simulink library "ddm"  (R2021b)
settings: Solver=VariableStepAuto  StartTime=0.0  StopTime=10.0  RelTol=1e-3
undefined symbols (not defined in the file or in its folder): ENUM_ADASACCSTA_ERROR, ENUM_ADASACCSTA_OFF, ENUM_ADASACCSTA_STANDBY, ENUM_ADASISASTA_OFF, ENUM_ALLOWMOV_ALLOWREADY, ENUM_APS, ENUM_BRKSTA_ERROR, ENUM_BRKSTA_OFF, ENUM_BRKSTA_ON, ENUM_CHGPREACTERRSTA_OBCPRE, ENUM_DCDCFAULTSTA_ANYFAULTLV1, ENUM_DCDCFAULTSTA_ANYFAULTLV2, ENUM_DRIVETRAIN_AWD, ENUM_DRIVETRAIN_FWD, ENUM_DRIVETRAIN_RWD, ENUM_DRSEATSTA_INVALID, ENUM_EDUDRTSTA_NORMAL, ENUM_EPBSTA_APPLIED, ENUM_EPBSTA_RELEASED, ENUM_HVBATTREADYPRE_READY, ENUM_MCUWARN_LV0, ENUM_MCUWARN_LV1, ENUM_MCUWARN_LV2, ENUM_MCUWARN_LV3, ENUM_MCUWARN_NOERROR, ENUM_OBCFAULTSTA_ANYFAULT, ENUM_PAS_R2F2, ENUM_PDFAULT_BATTPDFAIL, ENUM_PDFAULT_DCDCDISABLE, ENUM_PDFAULT_MCUDISABLE, ENUM_PDFAULT_MCUDISCHRG, ENUM_POWERSTA_OFF, ENUM_POWERSTA_ON, ENUM_POWERSTA_READY, ENUM_POWERSTA_STANDBY, ENUM_PRESSINDI_LOW, ENUM_PUFAULT_BATTUPFAIL, ENUM_PUFAULT_DCDCENABLEFAIL, ENUM_PUFAULT_PRECHRGCHKFAIL, ENUM_PUFAULT_SAFETYCHKFAIL, ENUM_PUSTATE_COMPLETED, ENUM_PWRSTASW_OFF, ENUM_PWRSTASW_OFFA, ENUM_PWRSTASW_OFFCHVCHRG, ENUM_PWRSTASW_OFFCLVCHRG, ENUM_PWRSTASW_ON, ENUM_PWRSTASW_ONHVCHRG, ENUM_PWRSTASW_READY, ENUM_PWRSTASW_STANDBY, ENUM_RANGESTA_12IN, ENUM_RANGESTA_12OUT, ENUM_SHIFTCOMMAND_D, ENUM_SHIFTCOMMAND_N, ENUM_SHIFTCOMMAND_P, ENUM_SHIFTCOMMAND_R, ENUM_ZONEMALFUNLV_1ST, ENUM_ZONEMALFUNLV_2ND, ENUM_ZONEMALFUNLV_3RD, ENUM_ZONEMALFUNLV_4TH, ENUM_ZONESPDCTRLMODE_ACC ... (+832)
libraries: hcu_lib x738, $bdroot x26, simulink x7
(part 12 of 25)

== system ddm/DDM/DDM/VMC_DDM/FCM5 ==
  task_time_s : Inport
  VDDM_FCM5NoCom_flg : Inport  Port=2
  VDDM_FCM5CSErr_flg : Inport  Port=3
  No_CAN_BUS_OFF : Inport  Port=4
  VPMM_PowerSta_enum : Inport  Port=5
  VINP_ADASISASta_enum : Inport  Port=6
  DTC_clear_request : Inport  Port=7
  Constant18 : Constant  Commented=on  Value=TRUE
  Constant21 : Constant  Commented=on  Value=FALSE
  "FCM5 Checksum Error " : Subsystem
  FCM5 Lost Com : Subsystem
  "FCM5 Rolling Count Error " : Subsystem  Commented=on
  From11 : From  Commented=on  GotoTag=DTC_clear_request
  From15 : From  Commented=on  GotoTag=VDDM_FCM5NoComCFS_flg
  From16 : From  Commented=on  GotoTag=VDDM_FCM5RCErrCFS_flg
  From17 : From  Commented=on  GotoTag=VDDM_FCM5CSErrCFS_flg
  From19 : From  Commented=on  GotoTag=task_time_s
  From21 : From  Commented=on  GotoTag=VDDM_FCM5RCErrCFS_flg
  From22 : From  Commented=on  GotoTag=VDDM_FCM5RCErrDFS_flg
  From23 : From  Commented=on  GotoTag=VDDM_VCUISAErr_flg
  From31 : From  Commented=on  GotoTag=VINP_ADASISASta_enum
  From6 : From  Commented=on  GotoTag=VDDM_FCM5NoComCFS_flg
  From7 : From  Commented=on  GotoTag=VDDM_FCM5RCErr_flg
  From8 : From  Commented=on  GotoTag=No_CAN_BUS_OFF
  From9 : From  Commented=on  GotoTag=VPMM_PowerSta_enum
  Goto11 : Goto  Commented=on  GotoTag=VDDM_VCUISAErr_flg
  Goto12 : Goto  Commented=on  GotoTag=VDDM_FCM5RCErr_flg
  Goto7 : Goto  Commented=on  GotoTag=VDDM_FCM5RCErrCFS_flg
  Goto8 : Goto  Commented=on  GotoTag=VDDM_FCM5RCErrDFS_flg
  Ground : Ground
  Logical Operator2 : Logic  Commented=on  Operator=OR  Inputs=3  AllPortsSameDT=off  OutDataTypeStr=boolean
  Switch : Switch  Commented=on  Criteria=u2 ~= 0
  Terminator : Terminator
  Terminator1 : Terminator
  Terminator2 : Terminator
  VDDM_FCM5NoComDFS_flg : Outport
  VDDM_FCM5NoComCFS_flg : Outport  Port=2
  VDDM_FCM5CSErrDFS_flg : Outport  Port=3
  VDDM_FCM5CSErrCFS_flg : Outport  Port=4
  VDDM_FCM5NoComDTC_raw32 : Outport  Port=5
  VDDM_FCM5CSErrDTC_raw32 : Outport  Port=6
  wires:
  VDDM_FCM5NoCom_flg/1 -> [VDDM_FCM5NoCom_flg]
  [VDDM_FCM5NoCom_flg] -> FCM5 Lost Com/2(VDDM_FCM5NoCom_flg)
  No_CAN_BUS_OFF/1 -> [No_CAN_BUS_OFF]
  VPMM_PowerSta_enum/1 -> [VPMM_PowerSta_enum]
  DTC_clear_request/1 -> [DTC_clear_request]
  [No_CAN_BUS_OFF] -> FCM5 Lost Com/3(No_CAN_BUS_OFF)
  [VPMM_PowerSta_enum] -> FCM5 Lost Com/4(VPMM_PowerSta_enum)
  [DTC_clear_request] -> FCM5 Lost Com/6(DTC_clear_request)
  FCM5 Lost Com/2(VDDM_FCM5NoComCFS_flg) -> [VDDM_FCM5NoComCFS_flg]
  FCM5 Lost Com/1(VDDM_FCM5NoComDFS_flg) -> [VDDM_FCM5NoComDFS_flg]
  [VDDM_FCM5NoComDFS_flg] -> VDDM_FCM5NoComDFS_flg/1
  From6/1 -> "FCM5 Rolling Count Error "/4(VDDM_FCM5NoComCFS_flg)
  From7/1 -> "FCM5 Rolling Count Error "/2(VDDM_FCM5RCErr_flg)
  From8/1 -> "FCM5 Rolling Count Error "/3(No_CAN_BUS_OFF)
  From9/1 -> "FCM5 Rolling Count Error "/5(VPMM_PowerSta_enum)
  From11/1 -> "FCM5 Rolling Count Error "/7(DTC_clear_request)
  "FCM5 Rolling Count Error "/1(VDDM_FCM5RCErrDFS_flg) -> Goto8/1
  "FCM5 Rolling Count Error "/2(VDDM_FCM5RCErrCFS_flg) -> Goto7/1
  [VDDM_FCM5NoComCFS_flg] -> VDDM_FCM5NoComCFS_flg/1
  [VDDM_FCM5CSErrDFS_flg] -> VDDM_FCM5CSErrDFS_flg/1
  [VDDM_FCM5CSErrCFS_flg] -> VDDM_FCM5CSErrCFS_flg/1
  From21/1 -> Terminator1/1
  From22/1 -> Terminator/1
  Switch/1 -> Goto11/1
  From23/1 -> Terminator2/1
  Ground/1 -> Goto12/1
  VDDM_FCM5CSErr_flg/1 -> [VDDM_FCM5CSErr_flg]
  Constant18/1 -> Switch/1
  Constant21/1 -> Switch/3
  From15/1 -> Logical Operator2/1
  From16/1 -> Logical Operator2/2
  From17/1 -> Logical Operator2/3
  Logical Operator2/1 -> Switch/2
  [task_time_s] -> FCM5 Lost Com/1(task_time_s)
  task_time_s/1 -> [task_time_s]  "task_time_s"
  From19/1 -> "FCM5 Rolling Count Error "/1(task_time_s)
  [task_time_s] -> "FCM5 Checksum Error "/1(task_time_s)
  [DTC_clear_request] -> "FCM5 Checksum Error "/7(DTC_clear_request)
  [VPMM_PowerSta_enum] -> "FCM5 Checksum Error "/5(VPMM_PowerSta_enum)
  [No_CAN_BUS_OFF] -> "FCM5 Checksum Error "/3(No_CAN_BUS_OFF)
  [VDDM_FCM5CSErr_flg] -> "FCM5 Checksum Error "/2(VDDM_FCM5CSErr_flg)
  [VDDM_FCM5NoComCFS_flg] -> "FCM5 Checksum Error "/4(VDDM_FCM5NoComCFS_flg)
  "FCM5 Checksum Error "/1(VDDM_FCM5CSErrDFS_flg) -> [VDDM_FCM5CSErrDFS_flg]
  "FCM5 Checksum Error "/2(VDDM_FCM5CSErrCFS_flg) -> [VDDM_FCM5CSErrCFS_flg]
  [VINP_ADASISASta_enum] -> FCM5 Lost Com/5(VINP_ADASISASta_enum)
  VINP_ADASISASta_enum/1 -> [VINP_ADASISASta_enum]
  From31/1 -> "FCM5 Rolling Count Error "/6(VINP_ADASISASta_enum)
  [VINP_ADASISASta_enum] -> "FCM5 Checksum Error "/6(VINP_ADASISASta_enum)
  FCM5 Lost Com/3(VDDM_FCM5NoComDTC_raw32) -> [VDDM_FCM5NoComDTC_raw32]
  "FCM5 Checksum Error "/3(VDDM_FCM5CSErrDTC_raw32) -> [VDDM_FCM5CSErrDTC_raw32]
  [VDDM_FCM5NoComDTC_raw32] -> VDDM_FCM5NoComDTC_raw32/1
  [VDDM_FCM5CSErrDTC_raw32] -> VDDM_FCM5CSErrDTC_raw32/1

== system ddm/DDM/DDM/VMC_DDM/FCMACC Signal Error ==
  task_time_s : Inport
  VDDM_FCM4NoComCFS_flg : Inport  Port=2
  VDDM_FCM4CSErrCFS_flg : Inport  Port=3
  No_CAN_BUS_OFF : Inport  Port=4
  VPMM_PowerSta_enum : Inport  Port=5
  VINP_ADASACCSta_enum : Inport  Port=6
  DTC_clear_request : Inport  Port=7
  "FCMACC Signal Error " : Subsystem
  From5 : From  Commented=on  GotoTag=VDDM_FCMACCSigErrDFS_flg
  Terminator : Terminator
  VDDM_FCMACCSigErrCFS_flg : Outport
  VDDM_FCMACCSigErrDetDTC_raw32 : Outport  Port=2
  wires:
  VDDM_FCM4CSErrCFS_flg/1 -> [VDDM_FCM4CSErrCFS_flg]
  [VDDM_FCMACCSigErrCFS_flg] -> VDDM_FCMACCSigErrCFS_flg/1
  From5/1 -> Terminator/1
  "FCMACC Signal Error "/1(VDDM_FCMACCSigErrCFS_flg) -> [VDDM_FCMACCSigErrCFS_flg]
  DTC_clear_request/1 -> [DTC_clear_request]
  VPMM_PowerSta_enum/1 -> [VPMM_PowerSta_enum]
  No_CAN_BUS_OFF/1 -> [No_CAN_BUS_OFF]
  VDDM_FCM4NoComCFS_flg/1 -> [VDDM_FCM4NoComCFS_flg]
  [No_CAN_BUS_OFF] -> "FCMACC Signal Error "/4(No_CAN_BUS_OFF)
  [VPMM_PowerSta_enum] -> "FCMACC Signal Error "/5(VPMM_PowerSta_enum)
  [DTC_clear_request] -> "FCMACC Signal Error "/7(DTC_clear_request)
  task_time_s/1 -> [task_time_s]  "task_time_s"
  [task_time_s] -> "FCMACC Signal Error "/1(task_time_s)
  [VDDM_FCM4NoComCFS_flg] -> "FCMACC Signal Error "/2(VDDM_FCM4NoComCFS_flg)
  [VDDM_FCM4CSErrCFS_flg] -> "FCMACC Signal Error "/3(VDDM_FCM4CSErrCFS_flg)
  VINP_ADASACCSta_enum/1 -> [VINP_ADASACCSta_enum]
  [VINP_ADASACCSta_enum] -> "FCMACC Signal Error "/6(VINP_ADASACCSta_enum)
  "FCMACC Signal Error "/2(VDDM_FCMACCSigErrDetDTC_raw32) -> [VDDM_FCMACCSigErrDetDTC_raw32]
  [VDDM_FCMACCSigErrDetDTC_raw32] -> VDDM_FCMACCSigErrDetDTC_raw32/1

== system ddm/DDM/DDM/VMC_DDM/ISA Malfunction  ==
  task_time_s : Inport
  VDDM_BMSSigErrCFS_flg : Inport  Port=2
  VDDM_FrMCUSigErrCFS_flg : Inport  Port=3
  VDDM_RrMCUSigErrCFS_flg : Inport  Port=4
  VDDM_CCUSigErrCFS_flg : Inport  Port=5
  VDDM_FCM3NoComCFS_flg : Inport  Port=6
  VDDM_FCM3RCErrCFS_flg : Inport  Port=7
  VDDM_FCM3CSErrCFS_flg : Inport  Port=8
  VDDM_FCM5NoComCFS_flg : Inport  Port=9
  VDDM_FCM5CSErrCFS_flg : Inport  Port=10
  VDDM_ZoneSCPNoComCFS_flg : Inport  Port=11
  VDDM_MCUR1NoComCFS_flg : Inport  Port=12
  VDDM_MCUR1RCErrCFS_flg : Inport  Port=13
  VDDM_MCUR1CSErrCFS_flg : Inport  Port=14
  VDDM_MCUF1NoComCFS_flg : Inport  Port=15
  VDDM_MCUF1RCErrCFS_flg : Inport  Port=16
  VDDM_MCUF1CSErrCFS_flg : Inport  Port=17
  VDDM_ESC7NoComCFS_flg : Inport  Port=18
  VDDM_ESC7RCErrCFS_flg : Inport  Port=19
  VDDM_ESC7CSErrCFS_flg : Inport  Port=20
  VDDM_ESC1NoComCFS_flg : Inport  Port=21
  VDDM_ESC1RCErrCFS_flg : Inport  Port=22
  VDDM_ESC1CSErrCFS_flg : Inport  Port=23
  VDDM_ESC5NoComCFS_flg : Inport  Port=24
  VDDM_ESC5RCErrCFS_flg : Inport  Port=25
  VDDM_ESC5CSErrCFS_flg : Inport  Port=26
  No_CAN1_BUS_OFF : Inport  Port=27
  No_CAN3_BUS_OFF : Inport  Port=28
  No_CAN4_BUS_OFF : Inport  Port=29
  VPMM_PowerSta_enum : Inport  Port=30
  VINP_ZoneSpdCtrlMode_enum : Inport  Port=31
  DTC_clear_request : Inport  Port=32
  From5 : From  Commented=on  GotoTag=VDDM_ISAMalfuncDFS_flg
  ISA Malfunction : Subsystem
  Terminator : Terminator
  VDDM_ISAMalfuncCFS_flg : Outport
  VDDM_ISAMalfuncDetDTC_raw32 : Outport  Port=2
  wires:
  VDDM_BMSSigErrCFS_flg/1 -> [VDDM_BMSSigErrCFS_flg]
  [VDDM_ISAMalfuncCFS_flg] -> VDDM_ISAMalfuncCFS_flg/1
  From5/1 -> Terminator/1
  ISA Malfunction/1(VDDM_ISAMalfuncCFS_flg) -> [VDDM_ISAMalfuncCFS_flg]
  VPMM_PowerSta_enum/1 -> [VPMM_PowerSta_enum]
  No_CAN1_BUS_OFF/1 -> [No_CAN1_BUS_OFF]
  VINP_ZoneSpdCtrlMode_enum/1 -> [VINP_ZoneSpdCtrlMode_enum]
  task_time_s/1 -> [task_time_s]  "task_time_s"
  VDDM_FrMCUSigErrCFS_flg/1 -> [VDDM_FrMCUSigErrCFS_flg]
  VDDM_RrMCUSigErrCFS_flg/1 -> [VDDM_RrMCUSigErrCFS_flg]
  VDDM_CCUSigErrCFS_flg/1 -> [VDDM_CCUSigErrCFS_flg]
  VDDM_ZoneSCPNoComCFS_flg/1 -> [VDDM_ZoneSCPNoComCFS_flg]
  VDDM_ESC7CSErrCFS_flg/1 -> [VDDM_ESC7CSErrCFS_flg]
  VDDM_ESC7RCErrCFS_flg/1 -> [VDDM_ESC7RCErrCFS_flg]
  VDDM_ESC7NoComCFS_flg/1 -> [VDDM_ESC7NoComCFS_flg]
  VDDM_ESC1NoComCFS_flg/1 -> [VDDM_ESC1NoComCFS_flg]
  VDDM_ESC1RCErrCFS_flg/1 -> [VDDM_ESC1RCErrCFS_flg]
  VDDM_ESC1CSErrCFS_flg/1 -> [VDDM_ESC1CSErrCFS_flg]
  VDDM_MCUF1CSErrCFS_flg/1 -> [VDDM_MCUF1CSErrCFS_flg]
  VDDM_MCUF1RCErrCFS_flg/1 -> [VDDM_MCUF1RCErrCFS_flg]
  VDDM_MCUF1NoComCFS_flg/1 -> [VDDM_MCUF1NoComCFS_flg]
  VDDM_MCUR1NoComCFS_flg/1 -> [VDDM_MCUR1NoComCFS_flg]
  VDDM_MCUR1RCErrCFS_flg/1 -> [VDDM_MCUR1RCErrCFS_flg]
  VDDM_MCUR1CSErrCFS_flg/1 -> [VDDM_MCUR1CSErrCFS_flg]
  VDDM_ESC5CSErrCFS_flg/1 -> [VDDM_ESC5CSErrCFS_flg]
  VDDM_ESC5RCErrCFS_flg/1 -> [VDDM_ESC5RCErrCFS_flg]
  VDDM_ESC5NoComCFS_flg/1 -> [VDDM_ESC5NoComCFS_flg]
  No_CAN3_BUS_OFF/1 -> [No_CAN3_BUS_OFF]
  No_CAN4_BUS_OFF/1 -> [No_CAN4_BUS_OFF]
  DTC_clear_request/1 -> [DTC_clear_request]
  [task_time_s] -> ISA Malfunction/1(task_time_s)
  [VDDM_BMSSigErrCFS_flg] -> ISA Malfunction/2(VDDM_BMSSigErrCFS_flg)
  [VDDM_FrMCUSigErrCFS_flg] -> ISA Malfunction/3(VDDM_FrMCUSigErrCFS_flg)
  [VDDM_RrMCUSigErrCFS_flg] -> ISA Malfunction/4(VDDM_RrMCUSigErrCFS_flg)
  [VDDM_CCUSigErrCFS_flg] -> ISA Malfunction/5(VDDM_CCUSigErrCFS_flg)
  [VDDM_FCM3NoComCFS_flg] -> ISA Malfunction/6(VDDM_FCM3NoComCFS_flg)
  [VDDM_FCM3RCErrCFS_flg] -> ISA Malfunction/7(VDDM_FCM3RCErrCFS_flg)
  [VDDM_FCM3CSErrCFS_flg] -> ISA Malfunction/8(VDDM_FCM3CSErrCFS_flg)
  [VDDM_FCM5NoComCFS_flg] -> ISA Malfunction/9(VDDM_FCM5NoComCFS_flg)
  [VDDM_FCM5CSErrCFS_flg] -> ISA Malfunction/10(VDDM_FCM5CSErrCFS_flg)
  [VDDM_ZoneSCPNoComCFS_flg] -> ISA Malfunction/11(VDDM_ZoneSCPNoComCFS_flg)
  [VDDM_MCUR1NoComCFS_flg] -> ISA Malfunction/12(VDDM_MCUR1NoComCFS_flg)
  [VDDM_MCUR1RCErrCFS_flg] -> ISA Malfunction/13(VDDM_MCUR1RCErrCFS_flg)
  [VDDM_MCUR1CSErrCFS_flg] -> ISA Malfunction/14(VDDM_MCUR1CSErrCFS_flg)
  [VDDM_MCUF1NoComCFS_flg] -> ISA Malfunction/15(VDDM_MCUF1NoComCFS_flg)
  [VDDM_MCUF1RCErrCFS_flg] -> ISA Malfunction/16(VDDM_MCUF1RCErrCFS_flg)
  [VDDM_MCUF1CSErrCFS_flg] -> ISA Malfunction/17(VDDM_MCUF1CSErrCFS_flg)
  [VDDM_ESC7NoComCFS_flg] -> ISA Malfunction/18(VDDM_ESC7NoComCFS_flg)
  [VDDM_ESC7RCErrCFS_flg] -> ISA Malfunction/19(VDDM_ESC7RCErrCFS_flg)
  [VDDM_ESC7CSErrCFS_flg] -> ISA Malfunction/20(VDDM_ESC7CSErrCFS_flg)
  [VDDM_ESC1NoComCFS_flg] -> ISA Malfunction/21(VDDM_ESC1NoComCFS_flg)
  [VDDM_ESC1RCErrCFS_flg] -> ISA Malfunction/22(VDDM_ESC1RCErrCFS_flg)
  [VDDM_ESC1CSErrCFS_flg] -> ISA Malfunction/23(VDDM_ESC1CSErrCFS_flg)
  [VDDM_ESC5NoComCFS_flg] -> ISA Malfunction/24(VDDM_ESC5NoComCFS_flg)
  [VDDM_ESC5RCErrCFS_flg] -> ISA Malfunction/25(VDDM_ESC5RCErrCFS_flg)
  [VDDM_ESC5CSErrCFS_flg] -> ISA Malfunction/26(VDDM_ESC5CSErrCFS_flg)
  [No_CAN1_BUS_OFF] -> ISA Malfunction/27(No_CAN1_BUS_OFF)
  [No_CAN3_BUS_OFF] -> ISA Malfunction/28(No_CAN3_BUS_OFF)
  [No_CAN4_BUS_OFF] -> ISA Malfunction/29(No_CAN4_BUS_OFF)
  [VPMM_PowerSta_enum] -> ISA Malfunction/30(VPMM_PowerSta_enum)
  [VINP_ZoneSpdCtrlMode_enum] -> ISA Malfunction/31(VINP_ZoneSpdCtrlMode_enum)
  [DTC_clear_request] -> ISA Malfunction/32(DTC_clear_request)
  VDDM_FCM3CSErrCFS_flg/1 -> [VDDM_FCM3CSErrCFS_flg]
  VDDM_FCM3RCErrCFS_flg/1 -> [VDDM_FCM3RCErrCFS_flg]
  VDDM_FCM5NoComCFS_flg/1 -> [VDDM_FCM5NoComCFS_flg]
  VDDM_FCM5CSErrCFS_flg/1 -> [VDDM_FCM5CSErrCFS_flg]
  VDDM_FCM3NoComCFS_flg/1 -> [VDDM_FCM3NoComCFS_flg]
  ISA Malfunction/2(VDDM_ISAMalfuncDetDTC_raw32) -> [VDDM_ISAMalfuncDetDTC_raw32]
  [VDDM_ISAMalfuncDetDTC_raw32] -> VDDM_ISAMalfuncDetDTC_raw32/1

== system ddm/DDM/DDM/VMC_DDM/MCU_Fr Signal Error ==
  task_time_s : Inport
  VDDM_MCUF1NoComCFS_flg : Inport  Port=2
  VDDM_MCUF1RCErrCFS_flg : Inport  Port=3
  VDDM_MCUF1CSErrCFS_flg : Inport  Port=4
  No_CAN_BUS_OFF : Inport  Port=5
  VPMM_PowerSta_enum : Inport  Port=6
  VINP_MCUWarnF_enum : Inport  Port=7
  DTC_clear_request : Inport  Port=8
  From5 : From  Commented=on  GotoTag=VDDM_FrMCUSigErrDFS_flg
  "MCU_Fr Signal Error " : Subsystem
  Terminator : Terminator
  VDDM_FrMCUSigErrCFS_flg : Outport
  VDDM_FrMCUSigErrDetDTC_raw32 : Outport  Port=2
  wires:
  VDDM_MCUF1CSErrCFS_flg/1 -> [VDDM_MCUF1CSErrCFS_flg]
  VDDM_MCUF1RCErrCFS_flg/1 -> [VDDM_MCUF1RCErrCFS_flg]
  [VDDM_FrMCUSigErrCFS_flg] -> VDDM_FrMCUSigErrCFS_flg/1
  From5/1 -> Terminator/1
  "MCU_Fr Signal Error "/1(VDDM_FrMCUSigErrCFS_flg) -> [VDDM_FrMCUSigErrCFS_flg]
  DTC_clear_request/1 -> [DTC_clear_request]
  VPMM_PowerSta_enum/1 -> [VPMM_PowerSta_enum]
  No_CAN_BUS_OFF/1 -> [No_CAN_BUS_OFF]
  VDDM_MCUF1NoComCFS_flg/1 -> [VDDM_MCUF1NoComCFS_flg]
  VINP_MCUWarnF_enum/1 -> [VINP_MCUWarnF_enum]
  [VDDM_MCUF1NoComCFS_flg] -> "MCU_Fr Signal Error "/2(VDDM_MCUF1NoComCFS_flg)
  [VDDM_MCUF1RCErrCFS_flg] -> "MCU_Fr Signal Error "/3(VDDM_MCUF1RCErrCFS_flg)
  [VDDM_MCUF1CSErrCFS_flg] -> "MCU_Fr Signal Error "/4(VDDM_MCUF1CSErrCFS_flg)
  [No_CAN_BUS_OFF] -> "MCU_Fr Signal Error "/5(No_CAN_BUS_OFF)
  [VPMM_PowerSta_enum] -> "MCU_Fr Signal Error "/6(VPMM_PowerSta_enum)
  [VINP_MCUWarnF_enum] -> "MCU_Fr Signal Error "/7(VINP_MCUWarnF_enum)
  [DTC_clear_request] -> "MCU_Fr Signal Error "/8(DTC_clear_request)
  task_time_s/1 -> [task_time_s]  "task_time_s"
  [task_time_s] -> "MCU_Fr Signal Error "/1(task_time_s)
  "MCU_Fr Signal Error "/2(VDDM_FrMCUSigErrDetDTC_raw32) -> [VDDM_FrMCUSigErrDetDTC_raw32]
  [VDDM_FrMCUSigErrDetDTC_raw32] -> VDDM_FrMCUSigErrDetDTC_raw32/1

== system ddm/DDM/DDM/VMC_DDM/MCU_Rr Signal Error ==
  task_time_s : Inport
  VDDM_MCUF1NoComCFS_flg : Inport  Port=2
  VDDM_MCUF1RCErrCFS_flg : Inport  Port=3
  VDDM_MCUF1CSErrCFS_flg : Inport  Port=4
  No_CAN_BUS_OFF : Inport  Port=5
  VPMM_PowerSta_enum : Inport  Port=6
  VINP_MCUWarnR_enum : Inport  Port=7
  DTC_clear_request : Inport  Port=8
  From5 : From  Commented=on  GotoTag=VDDM_RrMCUSigErrDFS_flg
  "MCU_Rr Signal Error " : Subsystem
  Terminator : Terminator
  VDDM_RrMCUSigErrCFS_flg : Outport
  VDDM_RrMCUSigErrDetDTC_raw32 : Outport  Port=2
  wires:
  VDDM_MCUF1CSErrCFS_flg/1 -> [VDDM_MCUF1CSErrCFS_flg]
  VDDM_MCUF1RCErrCFS_flg/1 -> [VDDM_MCUF1RCErrCFS_flg]
  [VDDM_RrMCUSigErrCFS_flg] -> VDDM_RrMCUSigErrCFS_flg/1
  From5/1 -> Terminator/1
  "MCU_Rr Signal Error "/1(VDDM_RrMCUSigErrCFS_flg) -> [VDDM_RrMCUSigErrCFS_flg]
  DTC_clear_request/1 -> [DTC_clear_request]
  VPMM_PowerSta_enum/1 -> [VPMM_PowerSta_enum]
  No_CAN_BUS_OFF/1 -> [No_CAN_BUS_OFF]
  VDDM_MCUF1NoComCFS_flg/1 -> [VDDM_MCUF1NoComCFS_flg]
  VINP_MCUWarnR_enum/1 -> [VINP_MCUWarnR_enum]
  [VDDM_MCUF1NoComCFS_flg] -> "MCU_Rr Signal Error "/2(VDDM_MCUF1NoComCFS_flg)
  [VDDM_MCUF1RCErrCFS_flg] -> "MCU_Rr Signal Error "/3(VDDM_MCUF1RCErrCFS_flg)
  [VDDM_MCUF1CSErrCFS_flg] -> "MCU_Rr Signal Error "/4(VDDM_MCUF1CSErrCFS_flg)
  [No_CAN_BUS_OFF] -> "MCU_Rr Signal Error "/5(No_CAN_BUS_OFF)
  [VPMM_PowerSta_enum] -> "MCU_Rr Signal Error "/6(VPMM_PowerSta_enum)
  [VINP_MCUWarnR_enum] -> "MCU_Rr Signal Error "/7(VINP_MCUWarnR_enum)
  [DTC_clear_request] -> "MCU_Rr Signal Error "/8(DTC_clear_request)
  task_time_s/1 -> [task_time_s]  "task_time_s"
  [task_time_s] -> "MCU_Rr Signal Error "/1(task_time_s)
  "MCU_Rr Signal Error "/2(VDDM_RrMCUSigErrDetDTC_raw32) -> [VDDM_RrMCUSigErrDetDTC_raw32]
  [VDDM_RrMCUSigErrDetDTC_raw32] -> VDDM_RrMCUSigErrDetDTC_raw32/1

== system ddm/DDM/DDM/VMC_DDM/MSA Malfunction  ==
  task_time_s : Inport
  VDDM_BMSSigErrCFS_flg : Inport  Port=2
  VDDM_FrMCUSigErrCFS_flg : Inport  Port=3
  VDDM_RrMCUSigErrCFS_flg : Inport  Port=4
  VDDM_CCUSigErrCFS_flg : Inport  Port=5
  VDDM_ZoneSCPNoComCFS_flg : Inport  Port=6
  VDDM_MCUR1NoComCFS_flg : Inport  Port=7
  VDDM_MCUR1RCErrCFS_flg : Inport  Port=8
  VDDM_MCUR1CSErrCFS_flg : Inport  Port=9
  VDDM_MCUF1NoComCFS_flg : Inport  Port=10
  VDDM_MCUF1RCErrCFS_flg : Inport  Port=11
  VDDM_MCUF1CSErrCFS_flg : Inport  Port=12
  VDDM_ESC7NoComCFS_flg : Inport  Port=13
  VDDM_ESC7RCErrCFS_flg : Inport  Port=14
  VDDM_ESC7CSErrCFS_flg : Inport  Port=15
  VDDM_ESC1NoComCFS_flg : Inport  Port=16
  VDDM_ESC1RCErrCFS_flg : Inport  Port=17
  VDDM_ESC1CSErrCFS_flg : Inport  Port=18
  VDDM_ESC5NoComCFS_flg : Inport  Port=19
  VDDM_ESC5RCErrCFS_flg : Inport  Port=20
  VDDM_ESC5CSErrCFS_flg : Inport  Port=21
  No_CAN1_BUS_OFF : Inport  Port=22
  No_CAN3_BUS_OFF : Inport  Port=23
  No_CAN4_BUS_OFF : Inport  Port=24
  VPMM_PowerSta_enum : Inport  Port=25
  VINP_ZoneSpdCtrlMode_enum : Inport  Port=26
  DTC_clear_request : Inport  Port=27
  From5 : From  Commented=on  GotoTag=VDDM_MSAMalfuncDFS_flg
  MSA Malfunction : Subsystem
  Terminator : Terminator
  VDDM_MSAMalfuncCFS_flg : Outport
  VDDM_MSAMalfuncDetDTC_raw32 : Outport  Port=2
  wires:
  VDDM_BMSSigErrCFS_flg/1 -> [VDDM_BMSSigErrCFS_flg]
  [VDDM_MSAMalfuncCFS_flg] -> VDDM_MSAMalfuncCFS_flg/1
  From5/1 -> Terminator/1
  MSA Malfunction/1(VDDM_MSAMalfuncCFS_flg) -> [VDDM_MSAMalfuncCFS_flg]
  VPMM_PowerSta_enum/1 -> [VPMM_PowerSta_enum]
  No_CAN1_BUS_OFF/1 -> [No_CAN1_BUS_OFF]
  VINP_ZoneSpdCtrlMode_enum/1 -> [VINP_ZoneSpdCtrlMode_enum]
  task_time_s/1 -> [task_time_s]  "task_time_s"
  VDDM_FrMCUSigErrCFS_flg/1 -> [VDDM_FrMCUSigErrCFS_flg]
  VDDM_RrMCUSigErrCFS_flg/1 -> [VDDM_RrMCUSigErrCFS_flg]
  VDDM_CCUSigErrCFS_flg/1 -> [VDDM_CCUSigErrCFS_flg]
  VDDM_ZoneSCPNoComCFS_flg/1 -> [VDDM_ZoneSCPNoComCFS_flg]
  VDDM_ESC7CSErrCFS_flg/1 -> [VDDM_ESC7CSErrCFS_flg]
  VDDM_ESC7RCErrCFS_flg/1 -> [VDDM_ESC7RCErrCFS_flg]
  VDDM_ESC7NoComCFS_flg/1 -> [VDDM_ESC7NoComCFS_flg]
  VDDM_ESC1NoComCFS_flg/1 -> [VDDM_ESC1NoComCFS_flg]
  VDDM_ESC1RCErrCFS_flg/1 -> [VDDM_ESC1RCErrCFS_flg]
  VDDM_ESC1CSErrCFS_flg/1 -> [VDDM_ESC1CSErrCFS_flg]
  VDDM_MCUF1CSErrCFS_flg/1 -> [VDDM_MCUF1CSErrCFS_flg]
  VDDM_MCUF1RCErrCFS_flg/1 -> [VDDM_MCUF1RCErrCFS_flg]
  VDDM_MCUF1NoComCFS_flg/1 -> [VDDM_MCUF1NoComCFS_flg]
  VDDM_MCUR1NoComCFS_flg/1 -> [VDDM_MCUR1NoComCFS_flg]
  VDDM_MCUR1RCErrCFS_flg/1 -> [VDDM_MCUR1RCErrCFS_flg]
  VDDM_MCUR1CSErrCFS_flg/1 -> [VDDM_MCUR1CSErrCFS_flg]
  VDDM_ESC5CSErrCFS_flg/1 -> [VDDM_ESC5CSErrCFS_flg]
  VDDM_ESC5RCErrCFS_flg/1 -> [VDDM_ESC5RCErrCFS_flg]
  VDDM_ESC5NoComCFS_flg/1 -> [VDDM_ESC5NoComCFS_flg]
  No_CAN3_BUS_OFF/1 -> [No_CAN3_BUS_OFF]
  No_CAN4_BUS_OFF/1 -> [No_CAN4_BUS_OFF]
  DTC_clear_request/1 -> [DTC_clear_request]
  [task_time_s] -> MSA Malfunction/1(task_time_s)
  [VDDM_BMSSigErrCFS_flg] -> MSA Malfunction/2(VDDM_BMSSigErrCFS_flg)
  [VDDM_FrMCUSigErrCFS_flg] -> MSA Malfunction/3(VDDM_FrMCUSigErrCFS_flg)
  [VDDM_RrMCUSigErrCFS_flg] -> MSA Malfunction/4(VDDM_RrMCUSigErrCFS_flg)
  [VDDM_CCUSigErrCFS_flg] -> MSA Malfunction/5(VDDM_CCUSigErrCFS_flg)
  [VDDM_ZoneSCPNoComCFS_flg] -> MSA Malfunction/6(VDDM_ZoneSCPNoComCFS_flg)
  [VDDM_MCUR1NoComCFS_flg] -> MSA Malfunction/7(VDDM_MCUR1NoComCFS_flg)
  [VDDM_MCUR1RCErrCFS_flg] -> MSA Malfunction/8(VDDM_MCUR1RCErrCFS_flg)
  [VDDM_MCUR1CSErrCFS_flg] -> MSA Malfunction/9(VDDM_MCUR1CSErrCFS_flg)
  [VDDM_MCUF1NoComCFS_flg] -> MSA Malfunction/10(VDDM_MCUF1NoComCFS_flg)
  [VDDM_MCUF1RCErrCFS_flg] -> MSA Malfunction/11(VDDM_MCUF1RCErrCFS_flg)
  [VDDM_MCUF1CSErrCFS_flg] -> MSA Malfunction/12(VDDM_MCUF1CSErrCFS_flg)
  [VDDM_ESC7NoComCFS_flg] -> MSA Malfunction/13(VDDM_ESC7NoComCFS_flg)
  [VDDM_ESC7RCErrCFS_flg] -> MSA Malfunction/14(VDDM_ESC7RCErrCFS_flg)
  [VDDM_ESC7CSErrCFS_flg] -> MSA Malfunction/15(VDDM_ESC7CSErrCFS_flg)
  [VDDM_ESC1NoComCFS_flg] -> MSA Malfunction/16(VDDM_ESC1NoComCFS_flg)
  [VDDM_ESC1RCErrCFS_flg] -> MSA Malfunction/17(VDDM_ESC1RCErrCFS_flg)
  [VDDM_ESC1CSErrCFS_flg] -> MSA Malfunction/18(VDDM_ESC1CSErrCFS_flg)
  [VDDM_ESC5NoComCFS_flg] -> MSA Malfunction/19(VDDM_ESC5NoComCFS_flg)
  [VDDM_ESC5RCErrCFS_flg] -> MSA Malfunction/20(VDDM_ESC5RCErrCFS_flg)
  [VDDM_ESC5CSErrCFS_flg] -> MSA Malfunction/21(VDDM_ESC5CSErrCFS_flg)
  [No_CAN1_BUS_OFF] -> MSA Malfunction/22(No_CAN1_BUS_OFF)
  [No_CAN3_BUS_OFF] -> MSA Malfunction/23(No_CAN3_BUS_OFF)
  [No_CAN4_BUS_OFF] -> MSA Malfunction/24(No_CAN4_BUS_OFF)
  [VPMM_PowerSta_enum] -> MSA Malfunction/25(VPMM_PowerSta_enum)
  [VINP_ZoneSpdCtrlMode_enum] -> MSA Malfunction/26(VINP_ZoneSpdCtrlMode_enum)
  [DTC_clear_request] -> MSA Malfunction/27(DTC_clear_request)
  MSA Malfunction/2(VDDM_MSAMalfuncDetDTC_raw32) -> [VDDM_MSAMalfuncDetDTC_raw32]
  [VDDM_MSAMalfuncDetDTC_raw32] -> VDDM_MSAMalfuncDetDTC_raw32/1

== system ddm/DDM/DDM/VMC_DDM/ZoneSCP ==
  task_time_s : Inport
  VDDM_ZoneSCPNoCom_flg : Inport  Port=2
  No_CAN_BUS_OFF : Inport  Port=3
  VPMM_PowerSta_enum : Inport  Port=4
  VINP_VehSpeed_kph : Inport  Port=5
  DTC_clear_request : Inport  Port=6
  From30 : From  Commented=on  GotoTag=VDDM_VCUACCErr_flg
  Terminator : Terminator
  ZoneSCP Lost Com : Subsystem
  VDDM_ZoneSCPNoComDFS_flg : Outport
  VDDM_ZoneSCPNoComCFS_flg : Outport  Port=2
  VDDM_ZoneSCPNoComDTC_raw32 : Outport  Port=3
  wires:
  VDDM_ZoneSCPNoCom_flg/1 -> [VDDM_ZoneSCPNoCom_flg]
  [VDDM_ZoneSCPNoCom_flg] -> ZoneSCP Lost Com/2(VDDM_ZoneSCPNoCom_flg)
  No_CAN_BUS_OFF/1 -> [No_CAN_BUS_OFF]
  VPMM_PowerSta_enum/1 -> [VPMM_PowerSta_enum]
  VINP_VehSpeed_kph/1 -> [VINP_VehSpeed_kph]
  DTC_clear_request/1 -> [DTC_clear_request]
  [No_CAN_BUS_OFF] -> ZoneSCP Lost Com/3(No_CAN_BUS_OFF)
  [VPMM_PowerSta_enum] -> ZoneSCP Lost Com/4(VPMM_PowerSta_enum)
  [VINP_VehSpeed_kph] -> ZoneSCP Lost Com/5(VINP_VehSpeed_kph)
  [DTC_clear_request] -> ZoneSCP Lost Com/6(DTC_clear_request)
  ZoneSCP Lost Com/2(VDDM_ZoneSCPNoComCFS_flg) -> [VDDM_ZoneSCPNoComCFS_flg]
  ZoneSCP Lost Com/1(VDDM_ZoneSCPNoComDFS_flg) -> [VDDM_ZoneSCPNoComDFS_flg]
  [VDDM_ZoneSCPNoComDFS_flg] -> VDDM_ZoneSCPNoComDFS_flg/1
  [VDDM_ZoneSCPNoComCFS_flg] -> VDDM_ZoneSCPNoComCFS_flg/1
  From30/1 -> Terminator/1
  [task_time_s] -> ZoneSCP Lost Com/1(task_time_s)
  task_time_s/1 -> [task_time_s]  "task_time_s"
  ZoneSCP Lost Com/3(VDDM_ZoneSCPNoComDTC_raw32) -> [VDDM_ZoneSCPNoComDTC_raw32]
  [VDDM_ZoneSCPNoComDTC_raw32] -> VDDM_ZoneSCPNoComDTC_raw32/1

== system ddm/DDM/DDM/PMM/Brake switch signal abnormal/Brake switch signal abnormal ==
  note: Release Condition During Failure Detection
  note: Test Detection Criteria
  note: Fail Safe Operation During Failure Detection
  note: Release Condition After Failure Decision
  note: Diagnostics and Fault Handling
  note: Fail Safe Operation After Failure Decision
  note: Test Pass Criteria
  task_time_s : Inport
  VPMM_PowerSta_enum : Inport  Port=2
  VPMM_PwrStaSW_enum : Inport  Port=3
  BrkSWErr : Inport  Port=4
  BrkSWPass : Inport  Port=5
  DTC_clear_request : Inport  Port=6
  Constant11 : Constant  Value=KDDM_BrkSWErrPassSW_flg
  Constant15 : Constant  Value=KDDM_BrkSWErrCFSSW_flg
  Constant16 : Constant  Value=TRUE
  Constant19 : Constant  Value=ENUM_POWERSTA_OFF
  Constant{2,21,25,27} (4 alike) : Constant  Value=FALSE
  Constant20 : Constant  Value=KDDM_BrkSWErrDFSSW_flg
  Constant22 : Constant  Value=ENUM_PWRSTASW_ON
  Constant23 : Constant  Value=TRUE
  Constant24 : Constant  Value=TRUE
  Constant26 : Constant  Value=ENUM_PWRSTASW_READY
  Constant28 : Constant  Value=ENUM_PWRSTASW_ON
  Constant29 : Constant  Value=ENUM_PWRSTASW_ONHVCHRG
  Constant3 : Constant  Value=ENUM_PWRSTASW_READY
  Constant38 : Constant  Value=KDDM_BrkSWErrDetTO_s
  Constant39 : Constant  Value=ENUM_PWRSTASW_ONHVCHRG
  Constant4 : Constant  Value=KDDM_BrkSWErrPassTO_s
  Constant40 : Constant  Value=KDDM_BrkSWErrDTC_cnt
  Constant43 : Constant  Value=KDDM_BrkSWErrPassTO_s
  Constant44 : Constant  Value=KDDM_BrkSWErrDetSW_flg
  Constant5 : Constant  Value=KDDM_BrkSWErrDTC_cnt
  DTC_Couter : hcu_lib/Basic_Blocks/DTC_Couter
  DTC_Info : hcu_lib/Basic_Blocks/DTC_Info
  Data Type Conversion1 : DataTypeConversion  OutDataTypeStr=uint8
  Equal{,2,4..6,17..18} (7 alike) : RelationalOperator  Operator===  OutDataTypeStr=boolean  RndMeth=Simplest
  Equal3 : RelationalOperator  OutDataTypeStr=boolean  RndMeth=Simplest
  Logical Operator{12,15,18..19} (4 alike) : Logic  AllPortsSameDT=off  OutDataTypeStr=boolean
  Logical Operator2 : Logic  Operator=OR  Inputs=3  AllPortsSameDT=off  OutDataTypeStr=boolean
  Logical Operator3 : Logic  Operator=OR  AllPortsSameDT=off  OutDataTypeStr=boolean
  Logical Operator5 : Logic  Operator=OR  Inputs=3  AllPortsSameDT=off  OutDataTypeStr=boolean
  Logical Operator6 : Logic  Operator=NOT  AllPortsSameDT=off  OutDataTypeStr=boolean
  Logical Operator8 : Logic  Operator=OR  AllPortsSameDT=off  OutDataTypeStr=boolean
  Relay : Relay  OnSwitchValue=ONE_INT  OffSwitchValue=ZERO_INT
  SR_Latch1 : Subsystem  mask(SR_Latch){}
      mask help: SR latch function.
  SR_Latch3 : hcu_lib/Basic_Blocks/SR_Latch
  SR_Latch4 : hcu_lib/Basic_Blocks/SR_Latch
  Switch{,2,4..6} (5 alike) : Switch  Criteria=u2 ~= 0
  Test Detection Criteria : hcu_lib/Basic_Blocks/Test Detection Criteria
  Timer1 : hcu_lib/Basic_Blocks/Timer
  VDDM_BrkSWErrDTC_raw32 : Outport
  VDDM_EDriveSysErrBrake_flg : Outport  Port=2
  wires:
  VPMM_PowerSta_enum/1 -> [VPMM_PowerSta_enum]
  VPMM_PwrStaSW_enum/1 -> [VPMM_PwrStaSW_enum]
  task_time_s/1 -> [task_time_s]
  [VPMM_PwrStaSW_enum] -> Equal/1
  [VPMM_PowerSta_enum] -> Equal4/1
  Logical Operator12/1 -> [VDDM_BrkSWErrDFS_flg]
  DTC_Couter/1 -> SR_Latch4/1
  Logical Operator15/1 -> DTC_Couter/2
  DTC_Couter/2 -> Data Type Conversion1/1
  Constant11/1 -> Logical Operator15/2
  Logical Operator3/1 -> Logical Operator15/1
  Equal/1 -> Logical Operator2/2
  Logical Operator2/1 -> Switch5/2
  Constant24/1 -> Switch4/1
  Switch2/1 -> Logical Operator6/1, SR_Latch1/2(reset), Timer1/2
  Logical Operator19/1 -> DTC_Couter/1
  [VDDM_BrkSWErrCFSRls_flg] -> Logical Operator3/2
  Logical Operator6/1 -> Timer1/1
  Constant20/1 -> Logical Operator12/1
  Logical Operator18/1 -> [VDDM_BrkSWErrCFS_flg]
  Constant43/1 -> Timer1/4
  Switch4/1 -> [VDDM_BrkSWErrCFSRls_flg]
  Constant19/1 -> Equal4/2
  Constant5/1 -> DTC_Couter/3
  [VDDM_BrkSWErrPass_flg] -> Logical Operator3/1
  SR_Latch1/1(latched) -> [VDDM_BrkSWErrPass_flg]
  Switch/1 -> [VDDM_EDriveSysErrBrake_flg]
  [VDDM_BrkSWErrDTC_cnt] -> Relay/1
  Equal3/1 -> SR_Latch1/1(set)
  Constant16/1 -> Switch/1
  Constant25/1 -> Switch4/3
  [DTC_clear_request] -> Logical Operator8/2
  Constant40/1 -> Test Detection Criteria/3
  Data Type Conversion1/1 -> [VDDM_BrkSWErrDTC_cnt]  "VDDM_BrkSWErrDTC_cnt"
  Constant26/1 -> Equal/2
  Equal4/1 -> Logical Operator8/1
  Logical Operator8/1 -> Switch4/2
  [VDDM_BrkSWErrDet_flg] -> Logical Operator19/1
  Constant44/1 -> Logical Operator19/2
  [VDDM_BrkSWErrCFSRls_flg] -> SR_Latch4/2
  SR_Latch4/1 -> Logical Operator18/1
  Constant27/1 -> Switch5/3
  Relay/1 -> SR_Latch3/1
  SR_Latch3/1 -> Logical Operator12/2
  Constant23/1 -> Switch2/3
  [VDDM_BrkSWErrCFS_flg] -> Switch/2
  Test Detection Criteria/1 -> [VDDM_BrkSWErrDet_flg]  "VDDM_BrkSWErrDet_flg"
  Constant15/1 -> Logical Operator18/2
  Constant21/1 -> Switch/3
  Timer1/1 -> Equal3/1
  [task_time_s] -> Test Detection Criteria/2
  [VPMM_PwrStaSW_enum] -> Equal5/1
  Equal5/1 -> Logical Operator2/1
  [VPMM_PwrStaSW_enum] -> Equal6/1
  Equal6/1 -> Logical Operator2/3
  Constant28/1 -> Equal5/2
  Constant29/1 -> Equal6/2
  Equal17/1 -> Logical Operator5/1
  Constant22/1 -> Equal17/2
  Constant39/1 -> Equal18/2
  Equal2/1 -> Logical Operator5/2
  [VPMM_PwrStaSW_enum] -> Equal18/1
  Constant3/1 -> Equal2/2
  Equal18/1 -> Logical Operator5/3
  [VPMM_PwrStaSW_enum] -> Equal17/1
  [VPMM_PwrStaSW_enum] -> Equal2/1
  Logical Operator5/1 -> Switch2/2
  Constant4/1 -> Equal3/2
  [VDDM_EDriveSysErrBrake_flg] -> VDDM_EDriveSysErrBrake_flg/1
  DTC_clear_request/1 -> [DTC_clear_request]
  [task_time_s] -> Timer1/3
  DTC_Info/1 -> VDDM_BrkSWErrDTC_raw32/1  "VDDM_BrkSWErrDTC_raw32"
  [VDDM_BrkSWErrPass_flg] -> DTC_Info/2
  [VDDM_BrkSWErrCFS_flg] -> DTC_Info/3
  BrkSWErr/1 -> Switch5/1
  BrkSWPass/1 -> Switch2/1
  [VDDM_BrkSWErrCFS_flg] -> SR_Latch3/2
  [VDDM_BrkSWErrDet_flg] -> DTC_Info/1
  Constant38/1 -> Test Detection Criteria/4
  [DTC_clear_request] -> DTC_Info/4
  [DTC_clear_request] -> Switch6/2
  Switch6/1 -> Test Detection Criteria/1
  Switch5/1 -> Switch6/3
  Constant2/1 -> Switch6/1

== system ddm/DDM/DDM/PMM/Brake switch signal abnormal/Brake switch signal abnormal and no backup signal ==
  note: Fail Safe Operation After Failure Decision
  note: Test Pass Criteria
  note: Fail Safe Operation During Failure Detection
  note: Release Condition After Failure Decision
  note: Diagnostics and Fault Handling
  note: Test Detection Criteria
  note: Release Condition During Failure Detection
  task_time_s : Inport
  VPMM_PowerSta_enum : Inport  Port=2
  VPMM_PwrStaSW_enum : Inport  Port=3
  BrkSWNoBac : Inport  Port=4
  BrkSWPass : Inport  Port=5
  DTC_clear_request : Inport  Port=6
  Constant1 : Constant  Value=ENUM_PWRSTASW_OFFCLVCHRG
  Constant11 : Constant  Value=KDDM_BrkSWNoBacPassSW_flg
  Constant15 : Constant  Value=KDDM_BrkSWNoBacCFSSW_flg
  Constant16 : Constant  Value=TRUE
  Constant19 : Constant  Value=ENUM_POWERSTA_OFF
  Constant2 : Constant  Value=ENUM_PWRSTASW_OFFCLVCHRG
  Constant20 : Constant  Value=KDDM_BrkSWNoBacDFSSW_flg
  Constant{8,21,25,27} (4 alike) : Constant  Value=FALSE
  Constant23 : Constant  Value=TRUE
  Constant24 : Constant  Value=TRUE
  Constant26 : Constant  Value=ENUM_PWRSTASW_OFFCHVCHRG
  Constant28 : Constant  Value=ENUM_PWRSTASW_ON
  Constant29 : Constant  Value=ENUM_PWRSTASW_ONHVCHRG
  Constant3 : Constant  Value=ENUM_PWRSTASW_OFFCHVCHRG
  Constant38 : Constant  Value=KDDM_BrkSWNoBacDetTO_s
  Constant4 : Constant  Value=KDDM_BrkSWNoBacPassTO_s
  Constant40 : Constant  Value=KDDM_BrkSWNoBacDTC_cnt
  Constant43 : Constant  Value=KDDM_BrkSWNoBacPassTO_s
  Constant44 : Constant  Value=KDDM_BrkSWNoBacDetSW_flg
  Constant5 : Constant  Value=KDDM_BrkSWNoBacDTC_cnt
  Constant6 : Constant  Value=ENUM_PWRSTASW_ON
  Constant7 : Constant  Value=ENUM_PWRSTASW_ONHVCHRG
  DTC_Couter : hcu_lib/Basic_Blocks/DTC_Couter
  DTC_Info : hcu_lib/Basic_Blocks/DTC_Info
  Data Type Conversion1 : DataTypeConversion  OutDataTypeStr=uint8
  Equal{,1..2,4..6,13..14,17} (9 alike) : RelationalOperator  Operator===  OutDataTypeStr=boolean  RndMeth=Simplest
  Equal3 : RelationalOperator  OutDataTypeStr=boolean  RndMeth=Simplest
  Logical Operator{12,15,18..19} (4 alike) : Logic  AllPortsSameDT=off  OutDataTypeStr=boolean
  Logical Operator2 : Logic  Operator=OR  Inputs=4  AllPortsSameDT=off  OutDataTypeStr=boolean
  Logical Operator3 : Logic  Operator=OR  AllPortsSameDT=off  OutDataTypeStr=boolean
  Logical Operator5 : Logic  Operator=OR  Inputs=4  AllPortsSameDT=off  OutDataTypeStr=boolean
  Logical Operator6 : Logic  Operator=NOT  AllPortsSameDT=off  OutDataTypeStr=boolean
  Logical Operator8 : Logic  Operator=OR  AllPortsSameDT=off  OutDataTypeStr=boolean
  Relay : Relay  OnSwitchValue=ONE_INT  OffSwitchValue=ZERO_INT
  SR_Latch1 : Subsystem  mask(SR_Latch){}
      mask help: SR latch function.
  SR_Latch3 : hcu_lib/Basic_Blocks/SR_Latch
  SR_Latch4 : hcu_lib/Basic_Blocks/SR_Latch
  Switch{,2,4..6} (5 alike) : Switch  Criteria=u2 ~= 0
  Test Detection Criteria : hcu_lib/Basic_Blocks/Test Detection Criteria
  Timer1 : hcu_lib/Basic_Blocks/Timer
  VDDM_BrkSWNoBacDTC_raw32 : Outport
  VDDM_VCUBrkSWSta_flg : Outport  Port=2
  wires:
  task_time_s/1 -> [task_time_s]
  VPMM_PwrStaSW_enum/1 -> [VPMM_PwrStaSW_enum]
  VPMM_PowerSta_enum/1 -> [VPMM_PowerSta_enum]
  Logical Operator5/1 -> Switch2/2
  Constant28/1 -> Equal5/2
  Constant44/1 -> Logical Operator19/2
  Constant4/1 -> Equal3/2
  Constant29/1 -> Equal6/2
  Constant43/1 -> Timer1/4
  Timer1/1 -> Equal3/1
  [task_time_s] -> Test Detection Criteria/2
  Constant15/1 -> Logical Operator18/2
  Test Detection Criteria/1 -> [VDDM_BrkSWNoBacDet_flg]  "VDDM_BrkSWNoBacDet_flg"
  Constant21/1 -> Switch/3
  [VDDM_BrkSWNoBacCFS_flg] -> Switch/2
  Constant23/1 -> Switch2/3
  SR_Latch3/1 -> Logical Operator12/2
  Relay/1 -> SR_Latch3/1
  Constant27/1 -> Switch5/3
  [VDDM_BrkSWNoBacCFSRls_flg] -> SR_Latch4/2
  Equal4/1 -> Logical Operator8/1
  Logical Operator8/1 -> Switch4/2
  Data Type Conversion1/1 -> [VDDM_BrkSWNoBacDTC_cnt]  "VDDM_BrkSWNoBacDTC_cnt"
  [DTC_clear_request] -> Logical Operator8/2
  Constant25/1 -> Switch4/3
  Constant19/1 -> Equal4/2
  Constant5/1 -> DTC_Couter/3
  [VDDM_BrkSWNoBacPass_flg] -> Logical Operator3/1
  SR_Latch4/1 -> Logical Operator18/1
  [VDDM_BrkSWNoBacDTC_cnt] -> Relay/1
  Switch4/1 -> [VDDM_BrkSWNoBacCFSRls_flg]
  Equal3/1 -> SR_Latch1/1(set)
  Logical Operator6/1 -> Timer1/1
  [VDDM_BrkSWNoBacCFSRls_flg] -> Logical Operator3/2
  Constant20/1 -> Logical Operator12/1
  Constant16/1 -> Switch/1
  Constant24/1 -> Switch4/1
  Constant11/1 -> Logical Operator15/2
  [VDDM_BrkSWNoBacDet_flg] -> Logical Operator19/1
  Logical Operator3/1 -> Logical Operator15/1
  Switch2/1 -> Logical Operator6/1, SR_Latch1/2(reset), Timer1/2
  [VPMM_PowerSta_enum] -> Equal4/1
  SR_Latch1/1(latched) -> [VDDM_BrkSWNoBacPass_flg]
  Switch/1 -> [VDDM_VCUBrkSWSta_flg]
  Logical Operator15/1 -> DTC_Couter/2
  DTC_Couter/1 -> SR_Latch4/1
  [VPMM_PwrStaSW_enum] -> Equal/1
  Logical Operator2/1 -> Switch5/2
  Logical Operator19/1 -> DTC_Couter/1
  [VPMM_PwrStaSW_enum] -> Equal6/1
  [VPMM_PwrStaSW_enum] -> Equal5/1
  Constant40/1 -> Test Detection Criteria/3
  Logical Operator18/1 -> [VDDM_BrkSWNoBacCFS_flg]
  DTC_Couter/2 -> Data Type Conversion1/1
  Logical Operator12/1 -> [VDDM_BrkSWNoBacDFS_flg]
  Constant26/1 -> Equal/2
  [VPMM_PwrStaSW_enum] -> Equal1/1
  Constant1/1 -> Equal1/2
  Equal6/1 -> Logical Operator2/4
  Equal1/1 -> Logical Operator2/3
  Equal5/1 -> Logical Operator2/2
  Equal/1 -> Logical Operator2/1
  Equal2/1 -> Logical Operator5/1
  Equal14/1 -> Logical Operator5/2
  Equal13/1 -> Logical Operator5/3
  Equal17/1 -> Logical Operator5/4
  Constant2/1 -> Equal13/2
  [VPMM_PwrStaSW_enum] -> Equal13/1
  Constant3/1 -> Equal2/2
  [VPMM_PwrStaSW_enum] -> Equal14/1
  [VPMM_PwrStaSW_enum] -> Equal17/1
  [VPMM_PwrStaSW_enum] -> Equal2/1
  Constant7/1 -> Equal17/2
  Constant6/1 -> Equal14/2
  [VDDM_VCUBrkSWSta_flg] -> VDDM_VCUBrkSWSta_flg/1
  DTC_clear_request/1 -> [DTC_clear_request]
  [task_time_s] -> Timer1/3
  DTC_Info/1 -> VDDM_BrkSWNoBacDTC_raw32/1  "VDDM_BrkSWNoBacDTC_raw32"
  [VDDM_BrkSWNoBacPass_flg] -> DTC_Info/2
  [VDDM_BrkSWNoBacCFS_flg] -> DTC_Info/3
  BrkSWNoBac/1 -> Switch5/1
  BrkSWPass/1 -> Switch2/1
  [VDDM_BrkSWNoBacCFS_flg] -> SR_Latch3/2
  [VDDM_BrkSWNoBacDet_flg] -> DTC_Info/1
  Constant38/1 -> Test Detection Criteria/4
  [DTC_clear_request] -> DTC_Info/4
  [DTC_clear_request] -> Switch6/2
  Switch6/1 -> Test Detection Criteria/1
  Switch5/1 -> Switch6/3
  Constant8/1 -> Switch6/1

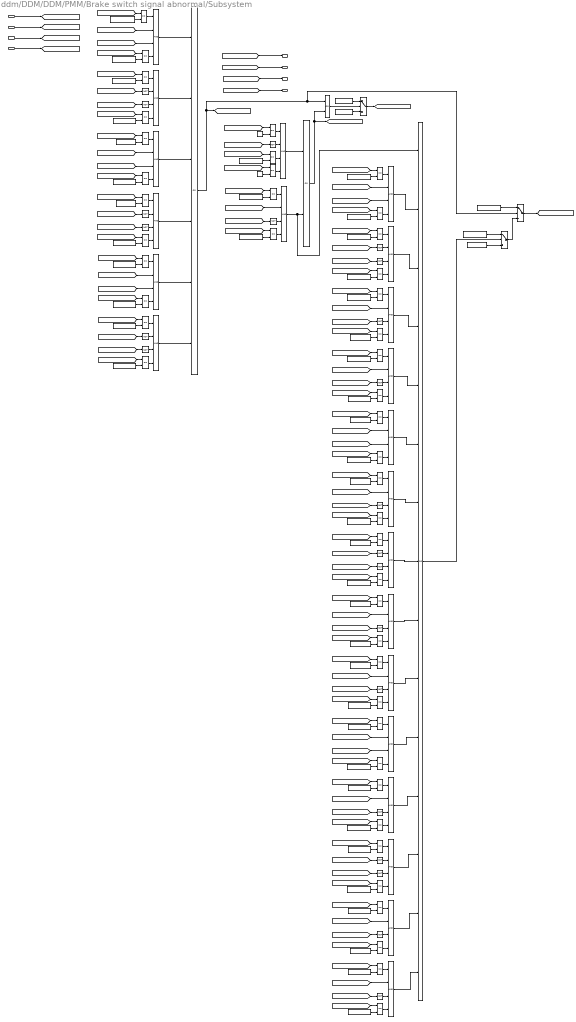
== system ddm/DDM/DDM/PMM/Brake switch signal abnormal/Subsystem ==
  note: 15
  note: 18
  note: 23
  note: 5
  note: 13
  note: 29
  note: 33
  note: 24
  note: 36
  note: 11
  note: 9
  note: 1
  note: 21
  note: 3
  note: 19
  note: 12
  note: 30
  note: 27
  note: 25
  note: 35
  note: 6
  note: 17
  VDDM_CANBSW2S_enum : Inport
  BrakeSW : Inport  Port=2
  Brake_Stop_Lamp : Inport  Port=3
  BrkPedalPos_enum : Inport  Port=4
  AND{,2..7,10,12..25} (22 alike) : Logic  Inputs=4  AllPortsSameDT=off  OutDataTypeStr=boolean
  AND1 : Logic  Operator=OR  Inputs=6  AllPortsSameDT=off  OutDataTypeStr=boolean
  AND11 : Logic  Operator=OR  Inputs=15  AllPortsSameDT=off  OutDataTypeStr=boolean
  AND8 : Logic  Operator=OR  AllPortsSameDT=off  OutDataTypeStr=boolean
  AND9 : Logic  Operator=OR  AllPortsSameDT=off  OutDataTypeStr=boolean
  Constant{1..10,15,17..18,23,29..30,32,46} (18 alike) : Constant  Value=ENUM_BRKSTA_ON
  Constant{16,19,21,25..28,31,38,47,50,53,55,57,59..61} (17 alike) : Constant  Value=ENUM_BRKSTA_ERROR
  Constant{20,22,24,33..34,39,41..45} (11 alike) : Constant  Value=ENUM_BRKSTA_OFF
  Constant35 : Constant  Value=FALSE
  Constant36 : Constant  Value=TRUE
  Constant37 : Constant  Value=0
  Constant40 : Constant  Value=0
  Equal{1..45} (45 alike) : RelationalOperator  Operator===  OutDataTypeStr=boolean  RndMeth=Simplest
  OR{,1..21} (22 alike) : Logic  Operator=NOT  AllPortsSameDT=off  OutDataTypeStr=boolean
  Switch6 : Switch  Criteria=u2 > Threshold
  Switch7 : Switch  Criteria=u2 > Threshold
  Switch8 : Switch  Criteria=u2 > Threshold
  BrkSWErr : Outport
  BrkSWNoBac : Outport  Port=2
  BrkSWPass : Outport  Port=3
  VDDM_BrakeSW_enum : Outport  Port=4
  wires:
  [BrkPedalPos_enum] -> Equal33/1
  Equal4/1 -> AND2/4
  OR2/1 -> AND4/2
  [BrakeSW] -> AND5/2
  Equal15/1 -> AND14/4
  Equal29/1 -> AND17/4
  Equal30/1 -> AND18/1
  Equal21/1 -> AND15/4
  OR/1 -> AND2/2
  OR15/1 -> AND20/3
  [Brake_Stop_Lamp] -> OR20/1
  [BrakeSW] -> AND12/2
  AND3/1 -> AND1/3
  [BrakeSW] -> OR17/1
  [BrakeSW] -> AND/2
  OR18/1 -> AND23/3
  Constant29/1 -> Equal39/2
  Constant22/1 -> Equal7/2
  OR5/1 -> AND6/3
  [BrakeSW] -> OR13/1
  [Brake_Stop_Lamp] -> OR18/1
  [Brake_Stop_Lamp] -> OR1/1
  Constant2/1 -> Equal22/2
  [VDDM_CANBSW2S_enum] -> Equal25/1
  [BrakeSW] -> OR2/1
  AND11/1 -> Switch7/2
  Constant46/1 -> Switch7/1
  [BrakeSW] -> AND15/2
  AND20/1 -> AND11/10
  AND18/1 -> AND11/8
  Constant27/1 -> Equal12/2
  AND23/1 -> AND11/13
  AND1/1 -> Switch8/2, AND9/1, [BrkSWNoBac]
  Constant59/1 -> Equal42/2
  [BrakeSW] -> OR6/1
  [BrkPedalPos_enum] -> Equal39/1
  AND21/1 -> AND11/11
  [BrkPedalPos_enum] -> Equal12/1
  [BrkPedalPos_enum] -> Equal19/1
  [VDDM_CANBSW2S_enum] -> Equal42/1
  [VDDM_CANBSW2S_enum] -> Equal32/1
  Constant23/1 -> Equal37/2
  OR4/1 -> AND6/2
  [VDDM_CANBSW2S_enum] -> Equal7/1
  OR20/1 -> AND25/3
  [BrakeSW] -> OR4/1
  Equal42/1 -> AND24/1
  Equal44/1 -> AND25/1
  [Brake_Stop_Lamp] -> OR11/1
  [BrkPedalPos_enum] -> Equal4/1
  Equal2/1 -> AND12/1
  Equal8/1 -> AND13/4
  [BrkPedalPos_enum] -> Equal18/1
  [Brake_Stop_Lamp] -> AND12/3
  OR10/1 -> AND15/3
  [VDDM_CANBSW2S_enum] -> Equal44/1
  Constant34/1 -> Equal28/2
  AND/1 -> AND1/1
  Constant35/1 -> Switch6/1
  AND24/1 -> AND11/14
  [BrkPedalPos_enum] -> Equal21/1
  [BrkPedalPos_enum] -> Equal13/1
  Switch6/1 -> [BrkSWErr]
  Equal1/1 -> AND/4
  Constant45/1 -> Switch7/3
  Equal38/1 -> AND22/1
  Equal11/1 -> AND5/1
  Equal3/1 -> AND13/1
  Equal40/1 -> AND23/1
  [Brake_Stop_Lamp] -> OR9/1
  [Brake_Stop_Lamp] -> OR21/1
  Constant47/1 -> Switch8/1
  OR21/1 -> AND7/3
  [BrakeSW] -> AND7/2
  Constant19/1 -> Equal4/2
  Equal45/1 -> AND25/4
  Constant17/1 -> Equal29/2
  Switch8/1 -> [VDDM_BrakeSW_enum]
  Equal32/1 -> AND19/1
  Constant41/1 -> Equal32/2
  [Brake_Stop_Lamp] -> OR16/1
  Constant24/1 -> Equal15/2
  [VDDM_CANBSW2S_enum] -> Equal36/1
  [Brake_Stop_Lamp] -> OR12/1
  OR12/1 -> AND18/3
  Equal41/1 -> AND23/4
  [BrakeSW] -> OR/1
  [VDDM_CANBSW2S_enum] -> Equal30/1
  AND7/1 -> AND11/1, AND8/2
  AND22/1 -> AND11/12
  Constant42/1 -> Equal33/2
  Equal6/1 -> AND3/4
  [Brake_Stop_Lamp] -> AND3/3
  [Brake_Stop_Lamp] -> OR5/1
  Constant10/1 -> Equal25/2
  [BrakeSW] -> OR7/1
  [VDDM_CANBSW2S_enum] -> Equal16/1
  Equal35/1 -> AND20/4
  Constant53/1 -> Equal36/2
  [BrakeSW] -> AND21/2
  [BrakeSW] -> AND22/2
  Constant20/1 -> Equal5/2
  Constant5/1 -> Equal2/2
  Constant60/1 -> Equal45/2
  [BrkPedalPos_enum] -> Equal37/1
  [Brake_Stop_Lamp] -> AND/3
  [VDDM_CANBSW2S_enum] -> Equal14/1
  Constant4/1 -> Equal18/2
  AND12/1 -> AND11/2
  [BrkPedalPos_enum] -> Equal1/1
  [BrakeSW] -> AND19/2
  [VDDM_CANBSW2S_enum] -> Equal40/1
  Constant36/1 -> Switch6/3
  Equal19/1 -> AND10/4
  [BrakeSW] -> AND20/2
  Constant1/1 -> Equal24/2
  AND8/1 -> [BrkSWPass], AND9/2
  OR9/1 -> AND14/3
  Equal10/1 -> AND4/4
  AND16/1 -> AND11/6
  OR6/1 -> AND10/2
  Constant55/1 -> Equal38/2
  [VDDM_CANBSW2S_enum] -> Equal11/1
  Constant57/1 -> Equal40/2
  Equal25/1 -> AND15/1
  Equal23/1 -> AND12/4
  AND13/1 -> AND11/3
  OR16/1 -> AND22/3
  Equal28/1 -> AND17/1
  Equal7/1 -> AND4/1
  [BrakeSW] -> AND3/2
  [BrkPedalPos_enum] -> Equal41/1
  Constant38/1 -> Equal21/2
  [BrakeSW] -> AND17/2
  [BrakeSW] -> AND14/2
  OR11/1 -> AND17/3
  AND10/1 -> AND8/1
  Constant6/1 -> Equal23/2
  Equal24/1 -> AND2/1
  AND15/1 -> AND11/5
  [BrakeSW] -> AND16/2
  [VDDM_CANBSW2S_enum] -> Equal26/1
  [BrkPedalPos_enum] -> Equal43/1
  OR14/1 -> AND19/3
  Equal27/1 -> AND16/4
  Constant15/1 -> Equal27/2
  AND19/1 -> AND11/9
  [BrkPedalPos_enum] -> Equal23/1
  [VDDM_CANBSW2S_enum] -> Equal34/1
  [BrkPedalPos_enum] -> Equal29/1
  Constant21/1 -> Equal6/2
  [BrkPedalPos_enum] -> Equal15/1
  Constant25/1 -> Equal10/2
  Equal37/1 -> AND21/4
  AND6/1 -> AND1/6
  AND5/1 -> AND1/5
  OR17/1 -> AND23/2
  Constant40/1 -> Equal19/2
  AND2/1 -> AND1/2
  Constant9/1 -> Equal9/2
  Constant18/1 -> Equal31/2
  Constant16/1 -> Equal1/2
  [VDDM_CANBSW2S_enum] -> Equal24/1
  Equal12/1 -> AND5/4
  Equal9/1 -> AND14/1
  Equal34/1 -> AND20/1
  Equal16/1 -> AND/1
  [BrakeSW] -> AND24/2
  OR7/1 -> AND13/2
  Equal26/1 -> AND16/1
  OR13/1 -> AND18/2
  Constant43/1 -> Equal34/2
  Constant30/1 -> Equal16/2
  AND17/1 -> AND11/7
  [Brake_Stop_Lamp] -> OR14/1
  [BrkPedalPos_enum] -> Equal8/1
  [VDDM_CANBSW2S_enum] -> Equal3/1
  [VDDM_CANBSW2S_enum] -> Equal28/1
  [VDDM_CANBSW2S_enum] -> Equal5/1
  Equal14/1 -> AND6/1
  Constant61/1 -> Equal44/2
  [BrkPedalPos_enum] -> Equal27/1
  Equal18/1 -> AND7/4
  [Brake_Stop_Lamp] -> AND16/3
  AND14/1 -> AND11/4
  [VDDM_CANBSW2S_enum] -> Equal17/1
  AND9/1 -> Switch6/2
  Equal13/1 -> AND6/4
  [VDDM_CANBSW2S_enum] -> Equal38/1
  [BrkPedalPos_enum] -> Equal31/1
  Equal31/1 -> AND18/4
  OR3/1 -> AND4/3
  [BrakeSW] -> AND25/2
  [BrkPedalPos_enum] -> Equal10/1
  OR19/1 -> AND24/3
  [Brake_Stop_Lamp] -> AND21/3
  Constant26/1 -> Equal11/2
  [Brake_Stop_Lamp] -> OR15/1
  [Brake_Stop_Lamp] -> OR3/1
  Equal5/1 -> AND3/1
  [VDDM_CANBSW2S_enum] -> Equal2/1
  [BrkPedalPos_enum] -> Equal6/1
  [Brake_Stop_Lamp] -> Equal22/1
  Equal20/1 -> AND10/1
  [VDDM_CANBSW2S_enum] -> Equal20/1
  [Brake_Stop_Lamp] -> OR19/1
  OR8/1 -> AND13/3
  Constant39/1 -> Equal30/2
  Constant44/1 -> Equal43/2
  Constant3/1 -> Equal17/2
  [Brake_Stop_Lamp] -> AND5/3
  Equal36/1 -> AND21/1
  Switch7/1 -> Switch8/3
  [BrkPedalPos_enum] -> Equal45/1
  Constant37/1 -> Equal20/2
  [VDDM_CANBSW2S_enum] -> Equal9/1
  Constant33/1 -> Equal26/2
  Equal43/1 -> AND24/4
  [BrkPedalPos_enum] -> Equal35/1
  Constant32/1 -> Equal41/2
  Constant50/1 -> Equal35/2
  Equal17/1 -> AND7/1
  Constant8/1 -> Equal8/2
  [Brake_Stop_Lamp] -> OR10/1
  [Brake_Stop_Lamp] -> OR8/1
  OR1/1 -> AND2/3
  Equal39/1 -> AND22/4
  Equal33/1 -> AND19/4
  Constant7/1 -> Equal3/2
  Equal22/1 -> AND10/3
  Constant31/1 -> Equal13/2
  AND25/1 -> AND11/15
  Constant28/1 -> Equal14/2
  AND4/1 -> AND1/4
  VDDM_CANBSW2S_enum/1 -> [VDDM_CANBSW2S_enum]
  BrakeSW/1 -> [BrakeSW]
  Brake_Stop_Lamp/1 -> [Brake_Stop_Lamp]
  BrkPedalPos_enum/1 -> [BrkPedalPos_enum]
  [BrkSWErr] -> BrkSWErr/1
  [BrkSWNoBac] -> BrkSWNoBac/1
  [BrkSWPass] -> BrkSWPass/1
  [VDDM_BrakeSW_enum] -> VDDM_BrakeSW_enum/1
